simulink library "RoverbotMotion"  (Simulink 6.4)
StartFcn:
  | ppo_start
StopFcn:
  | ppo_stop
settings Model: LastModifiedBy=Raza

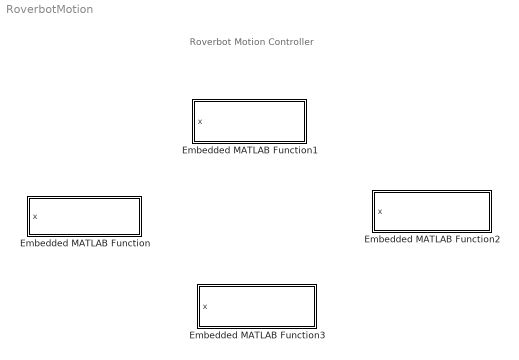
== system RoverbotMotion ==
  note: Roverbot Motion Controller
  Embedded MATLAB Function : Stateflow chart
  Embedded MATLAB Function1 : Stateflow chart
  Embedded MATLAB Function2 : Stateflow chart
  Embedded MATLAB Function3 : Stateflow chart

== matlab function Embedded MATLAB Function1 ==
  data: x input inherited
function GoStraight(x)
MoveForward(x);

== matlab function Embedded MATLAB Function ==
  data: x input inherited
function GoLeft(x)
MoveLeft(x);

== matlab function Embedded MATLAB Function2 ==
  data: x input inherited
function GoRight(x)
MoveRight(x);

== matlab function Embedded MATLAB Function3 ==
  data: x input inherited
function GoBackwards(x)
MoveBackward(x);
